simulink model "controller"  (R2024b)
settings: Solver=FixedStepAuto  StartTime=0.0  StopTime=10.0  FixedStep=1/100  RelTol=1e-3
undefined symbols (not defined in the file): MAX_TORQUE, MAX_TORQUE_REVERSE
settings Model: Creator=DAUIN-Win10  LastModifiedBy=siani
settings OptimizationCC: ReuseModelBlockBuffer=off
settings DebuggingCC: UnconnectedInputMsg=warning  UnconnectedOutputMsg=warning  UnconnectedLineMsg=warning
settings ModelReferenceCC: EnableRefExpFcnMdlSchedulingChecks=on
settings RTWCC: GPUComputeCapability=3.5  DLArmComputeVersion=19.05

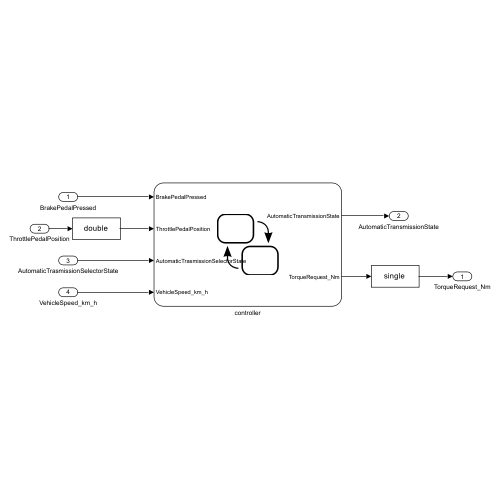
[thumbnail: Simulink's stored preview of the top-level diagram]
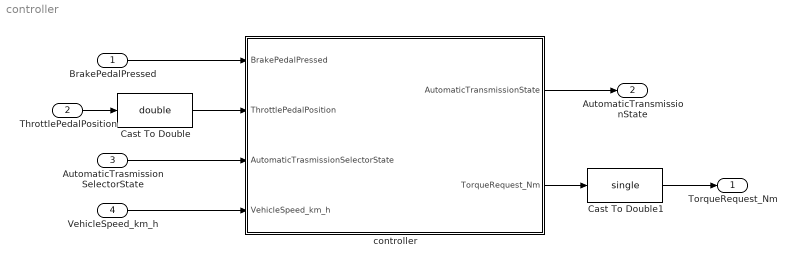
== system controller ==
  BrakePedalPressed : Inport  OutDataTypeStr=boolean
  ThrottlePedalPosition : Inport  Port=2  OutDataTypeStr=single
  AutomaticTrasmissionSelectorState : Inport  Port=3  OutDataTypeStr=Enum: TransmissionState
  VehicleSpeed_km_h : Inport  Port=4  OutDataTypeStr=single  Unit=km/h
  Cast To Double : DataTypeConversion  OutDataTypeStr=double  SaturateOnIntegerOverflow=off  RndMeth=Floor
  Cast To Double1 : DataTypeConversion  OutDataTypeStr=single  SaturateOnIntegerOverflow=off  RndMeth=Floor
  controller : Stateflow chart  TreatAsAtomicUnit=on
  TorqueRequest_Nm : Outport  OutDataTypeStr=single  Unit=N*m
  AutomaticTransmissionState : Outport  Port=2  OutDataTypeStr=Enum: TransmissionState
  wires:
  BrakePedalPressed/1 -> controller/1(BrakePedalPressed)
  VehicleSpeed_km_h/1 -> controller/4(VehicleSpeed_km_h)
  AutomaticTrasmissionSelectorState/1 -> controller/3(AutomaticTrasmissionSelectorState)
  ThrottlePedalPosition/1 -> Cast To Double/1
  controller/2(TorqueRequest_Nm) -> Cast To Double1/1
  controller/1(AutomaticTransmissionState) -> AutomaticTransmissionState/1
  Cast To Double/1 -> controller/2(ThrottlePedalPosition)
  Cast To Double1/1 -> TorqueRequest_Nm/1

== stateflow chart controller/controller ==
  state Park
    entry:
    AutomaticTransmissionState = TransmissionState.Park;
    during:
    TorqueRequest_Nm = 0;
  state Brake
    entry:
    AutomaticTransmissionState = TransmissionState.Brake;
    state Acceleration
      during:
      coeff = (3/2) * (ThrottlePedalPosition - 1/3);
      TorqueRequest_Nm = MAX_TORQUE  * coeff;
    state RegenerativeBraking
      during:
      coeff = 1 - 3 *ThrottlePedalPosition;
      TorqueRequest_Nm = - MAX_TORQUE * coeff;
    state EndBreakingRegion
      during:
      TorqueRequest_Nm =0;
    (default) -> Acceleration
    (junction 55) -> Acceleration
    EndBreakingRegion -> (junction 55) : [ThrottlePedalPosition > 1/3  || abs(VehicleSpeed_km_h)>0.2]
    Acceleration -> RegenerativeBraking : [ThrottlePedalPosition <= 1/3 && ThrottlePedalPosition >0]
    RegenerativeBraking -> Acceleration [order 1] : [ThrottlePedalPosition > 1/3 &&ThrottlePedalPosition <=1 ]
    RegenerativeBraking -> EndBreakingRegion [order 2] : [VehicleSpeed_km_h <= 0.2]
  state Drive
    entry:
    AutomaticTransmissionState = TransmissionState.Drive;
    during:
    TorqueRequest_Nm = ThrottlePedalPosition * MAX_TORQUE;
  state Neutral
    entry:
    AutomaticTransmissionState = TransmissionState.Neutral;
    during:
    TorqueRequest_Nm = 0;
  state Reverse
    entry:
    AutomaticTransmissionState = TransmissionState.Reverse;
    during:
    TorqueRequest_Nm = -ThrottlePedalPosition * MAX_TORQUE_REVERSE;
  (default) -> Park
  Neutral -> Park [order 1] : [AutomaticTrasmissionSelectorState == TransmissionState.Park && abs(VehicleSpeed_km_h) < 5 && BrakePedalPressed == 1]
  Park -> Neutral : [AutomaticTrasmissionSelectorState ~= TransmissionState.Park && BrakePedalPressed == 1]
  Brake -> Drive : [AutomaticTrasmissionSelectorState ~= TransmissionState.Brake]
  Drive -> Neutral [order 1] : [AutomaticTrasmissionSelectorState < TransmissionState.Drive]
  Neutral -> Reverse [order 2] : [AutomaticTrasmissionSelectorState == TransmissionState.Reverse && VehicleSpeed_km_h < 5 && BrakePedalPressed == 1]
  Drive -> Brake [order 2] : [AutomaticTrasmissionSelectorState == TransmissionState.Brake && ThrottlePedalPosition >= 1/3]
  Neutral -> Drive [order 3] : [AutomaticTrasmissionSelectorState >TransmissionState.Neutral && VehicleSpeed_km_h > -5 && BrakePedalPressed == 1]
  Reverse -> Neutral : [AutomaticTrasmissionSelectorState  ~= TransmissionState.Reverse]
  data: BrakePedalPressed input; ThrottlePedalPosition input; AutomaticTrasmissionSelectorState input Enum: TransmissionState; VehicleSpeed_km_h input; AutomaticTransmissionState output Enum: TransmissionState; TorqueRequest_Nm output; MAX_TORQUE parameter double; coeff local; MAX_TORQUE_REVERSE parameter double
